simulink model "iir_biquad"  (Simulink 10.0)
settings: Solver=FixedStepDiscrete  StartTime=0.0  StopTime=300  RelTol=1e-3
settings Model: Creator=moeller  LastModifiedBy=bhisma
settings SolverCC: AutoInsertRateTranBlk=on  InsertRTBMode=Always
settings DataIOCC: LimitDataPoints=on
settings OptimizationCC: BlockReduction=off  ConditionallyExecuteInputs=off  ExpressionDepthLimit=2147483647
settings DebuggingCC: SolverPrmCheckMsg=warning  MultiTaskCondExecSysMsg=warning  MultiTaskRateTransMsg=warning  FcnCallInpInsideContextMsg=warning  StateNameClashWarn=warning
settings GRTTargetCC: GeneratePreprocessorConditionals=Disable all
settings ConfigComp: CovExternalEMLEnable=off  CovSFcnEnable=off

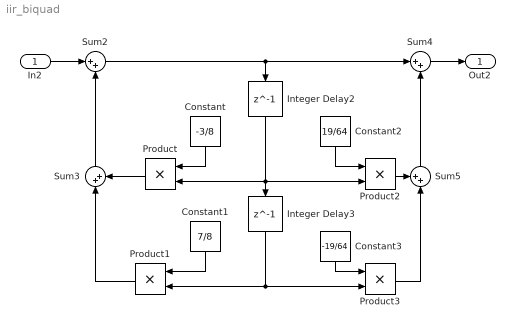
== system iir_biquad ==
  In2 : Inport
  Constant : Constant  Value=-3/8  OutDataTypeStr=fixdt(1,32,24)
  Constant1 : Constant  Value=7/8  OutDataTypeStr=fixdt(1,32,24)
  Constant2 : Constant  Value=19/64  OutDataTypeStr=fixdt(1,32,24)
  Constant3 : Constant  Value=-19/64  OutDataTypeStr=fixdt(1,32,24)
  Integer Delay2 : Delay  DelayLength=1  SampleTime=2
  Integer Delay3 : Delay  DelayLength=1  SampleTime=2
  Product{,1..3} (4 alike) : Product  OutDataTypeStr=fixdt(1,32,28)  RndMeth=Zero
  Sum2 : Sum  Inputs=|++  AccumDataTypeStr=fixdt(1,32,28)  OutDataTypeStr=fixdt(1,32,28)
  Sum3 : Sum  Inputs=|++  AccumDataTypeStr=fixdt(1,32,28)  OutDataTypeStr=fixdt(1,32,28)
  Sum4 : Sum  Inputs=|++  AccumDataTypeStr=fixdt(1,32,28)  OutDataTypeStr=fixdt(1,32,28)
  Sum5 : Sum  Inputs=++|  AccumDataTypeStr=fixdt(1,32,28)  OutDataTypeStr=fixdt(1,32,28)
  Out2 : Outport
  wires:
  Product3/1 -> Sum5/2
  Sum3/1 -> Sum2/2
  Product/1 -> Sum3/2
  Constant3/1 -> Product3/1
  Sum2/1 -> Sum4/1, Integer Delay2/1
  Constant1/1 -> Product1/1
  Product2/1 -> Sum5/1
  Sum5/1 -> Sum4/2
  Constant2/1 -> Product2/1
  Constant/1 -> Product/1
  Product1/1 -> Sum3/1
  In2/1 -> Sum2/1
  Sum4/1 -> Out2/1
  Integer Delay3/1 -> Product3/2, Product1/2
  Integer Delay2/1 -> Integer Delay3/1, Product2/2, Product/2
